simulink subsystem "Out_of_Plane_Model"  (R2025b)
settings: Solver=VariableStepAuto  StartTime=0.0  StopTime=10.0  RelTol=1e-3
undefined symbols (not defined in the file): AeroLiftCff, AeroLongDrgCff, AeroMotoEffctArea, AeroPitchMomentCff, AeroPitchMomentLngth, AeroRltWindAngVect, AeroSideFrcCff, AeroYawMomentCff, aMode, BrkFrntBrkActrBore, BrkFrntBrkActrPrsBpt, BrkFrntBrkPadMeanRadius, BrkFrntBrkTrqTbl, BrkFrntIntrnRadius, BrkFrntKinFricCff, BrkFrntPadNum, BrkFrntShoePinToDrumCntrDst, BrkFrntShoePinToFrcAppDst, BrkFrntShoePinToPadEndAng, BrkFrntShoePinToPadStartAng, BrkFrntStcFricCff, BrkFrntWhlSpdBpt, BrkRearBrkActrBore, BrkRearBrkActrPrsBpt, BrkRearBrkPadMeanRadius, BrkRearBrkTrqTbl, BrkRearIntrnRadius, BrkRearKinFricCff, BrkRearPadNum, BrkRearShoePinToDrumCntrDst, BrkRearShoePinToFrcAppDst, BrkRearShoePinToPadEndAng, BrkRearShoePinToPadStartAng, BrkRearStcFricCff, BrkRearWhlSpdBpt, CpRrVx0, CpRrVy0, CpRrY0, EnvAbsPrs, EnvAirTemp, FrkFrL0, FrmAng0, g, GasCnst, InitFrkLngth, InitMainFrmPitchAng, InitRearArmPitchAng, InitRearCntctPtchLatVel, InitRearCntctPtchLongVel, InitRearCntctPtchZ, InitYawAng, MotoFrmLngth, MotoFrmMass, MotoGrvty, MotoLatOfst, MotoLongOfst, MotoLowrFrntFrkMass, MotoPtchOfst, MotoRearArmLngth, MotoRearArmMass ... (+28)
libraries: sm_lib x309, nesl_utility_internal x158, nesl_utility x7, autolibsharedcoupling x6, vehdynlibtire x6, sharedtransform x4, shared6dof x1, matrix_library x1, vehdynlibeomcommon x1
(part 6 of 10)

== system Out_of_Plane_Model/Chassis, Tires, and Areo/Tire/Front Tire/Linear Front Simscape Tire/Simscape/apply forces and moments ==
  Fx : Inport
  Fy : Inport  Port=2
  Fz : Inport  Port=3
  Mxin : Inport  Port=4
  Mzin : Inport  Port=5
  External Force and Torque : sm_lib/Forces and Torques/External Force and Torque  EnableForceX=on  EnableForceY=on  EnableForceZ=on  EnableForce=off  ForceResolutionFrame=AttachedFrame  EnableTorqueX=on  EnableTorqueY=off  EnableTorqueZ=on  EnableTorque=off  TorqueResolutionFrame=AttachedFrame
  Simulink-PS Converter : nesl_utility_internal/Simulink-PS Converter  PhysicalDomain=network_engine_domain  SubClassName=ps_input  LeftPortType=input  RightPortType=output  PseudoPeriodic=off  Frequencies=[]  NoiseDistribution=none  NoiseParameters=[]  Unit=N  AffineConversion=off  FilteringAndDerivatives=zero  SimscapeFilterOrder=1  InputFilterTimeConstant=0.001  UdotUserProvided=1
  Simulink-PS Converter1 : nesl_utility_internal/Simulink-PS Converter  PhysicalDomain=network_engine_domain  SubClassName=ps_input  LeftPortType=input  RightPortType=output  PseudoPeriodic=off  Frequencies=[]  NoiseDistribution=none  NoiseParameters=[]  Unit=N  AffineConversion=off  FilteringAndDerivatives=zero  SimscapeFilterOrder=1  InputFilterTimeConstant=0.001  UdotUserProvided=1
  Simulink-PS Converter2 : nesl_utility_internal/Simulink-PS Converter  PhysicalDomain=network_engine_domain  SubClassName=ps_input  LeftPortType=input  RightPortType=output  PseudoPeriodic=off  Frequencies=[]  NoiseDistribution=none  NoiseParameters=[]  Unit=N  AffineConversion=off  FilteringAndDerivatives=zero  SimscapeFilterOrder=1  InputFilterTimeConstant=0.001  UdotUserProvided=1
  Simulink-PS Converter3 : nesl_utility_internal/Simulink-PS Converter  PhysicalDomain=network_engine_domain  SubClassName=ps_input  LeftPortType=input  RightPortType=output  PseudoPeriodic=off  Frequencies=[]  NoiseDistribution=none  NoiseParameters=[]  Unit=N*m  AffineConversion=off  FilteringAndDerivatives=zero  SimscapeFilterOrder=1  InputFilterTimeConstant=0.001  UdotUserProvided=1
  Simulink-PS Converter4 : nesl_utility_internal/Simulink-PS Converter  PhysicalDomain=network_engine_domain  SubClassName=ps_input  LeftPortType=input  RightPortType=output  PseudoPeriodic=off  Frequencies=[]  NoiseDistribution=none  NoiseParameters=[]  Unit=N*m  AffineConversion=off  FilteringAndDerivatives=zero  SimscapeFilterOrder=1  InputFilterTimeConstant=0.001  UdotUserProvided=1
  CP : PMIOPort  Side=Right
  wires:
  Fx/1 -> Simulink-PS Converter/1
  Fz/1 -> Simulink-PS Converter2/1
  Fy/1 -> Simulink-PS Converter1/1
  Mxin/1 -> Simulink-PS Converter3/1
  Mzin/1 -> Simulink-PS Converter4/1
  connections:
  External Force and Torque/LConn3 -- Simulink-PS Converter2/RConn1
  External Force and Torque/LConn1 -- Simulink-PS Converter/RConn1
  External Force and Torque/RConn1 -- CP/RConn1
  Simulink-PS Converter1/RConn1 -- External Force and Torque/LConn2
  External Force and Torque/LConn4 -- Simulink-PS Converter3/RConn1
  External Force and Torque/LConn5 -- Simulink-PS Converter4/RConn1

== system Out_of_Plane_Model/Chassis, Tires, and Areo/Tire/Rear Tire/Linear Rear Simscape Tire/Brake model/External ==
  MBrkin : Inport
  MBrk : Outport
  wires:
  MBrkin/1 -> MBrk/1

== system Out_of_Plane_Model/Chassis, Tires, and Areo/Tire/Rear Tire/Linear Rear Simscape Tire/Brake model/MW Brake ==
  BrkPrs : Inport
  Omega : Inport  Port=2
  Brakes : Subsystem  Variant=on  VariantControlMode=label  LabelModeActiveChoice=Disk  mask{aMode=aMode}
  Gain1 : Gain  Gain=4
  Product : Product
  Tanh : Trigonometry  Operator=tanh
  Unary Minus : UnaryMinus
  MBrk : Outport
  wires:
  BrkPrs/1 -> Brakes/1(BrkPrs)
  Unary Minus/1 -> MBrk/1
  Product/1 -> Unary Minus/1
  Omega/1 -> Brakes/2(Omega), Gain1/1
  Tanh/1 -> Product/2
  Brakes/1(MyBrk) -> Product/1
  Gain1/1 -> Tanh/1

== system Out_of_Plane_Model/Chassis, Tires, and Areo/Tire/Rear Tire/Linear Rear Simscape Tire/Contact model/External ==
  Fzin : Inport
  Fz : Outport
  wires:
  Fzin/1 -> Fz/1

== system Out_of_Plane_Model/Chassis, Tires, and Areo/Tire/Rear Tire/Linear Rear Simscape Tire/Contact model/Simple spring and damper ==
  rz : Inport
  pz : Inport  Port=2
  Add4 : Sum
  Gain17 : Gain  Gain=kz
  Gain18 : Gain  Gain=cz
  Unary Minus : UnaryMinus
  contact decision : Subsystem
  Fz : Outport
  wires:
  pz/1 -> Gain17/1, contact decision/1(pos)
  Gain17/1 -> Add4/1
  Add4/1 -> contact decision/2(Fpre)
  contact decision/1(F) -> Unary Minus/1
  Gain18/1 -> Add4/2
  rz/1 -> Gain18/1
  Unary Minus/1 -> Fz/1

== system Out_of_Plane_Model/Chassis, Tires, and Areo/Tire/Rear Tire/Linear Rear Simscape Tire/Friction model/External ==
  rx : Inport
  ry : Inport  Port=2
  rz : Inport  Port=3
  Omega : Inport  Port=4
  Fxin : Inport  Port=5
  Fyin : Inport  Port=6
  Mxin : Inport  Port=7
  Myin : Inport  Port=8
  Mzin : Inport  Port=9
  Calc. part Vertical load & SideSlipAngle : Subsystem
  Mux : Mux  Inputs=3
  SlipRatio : Subsystem
  Fx : Outport
  Fy : Outport  Port=2
  Kappa : Outport  Port=3
  Alpha : Outport  Port=4
  Mx : Outport  Port=5
  My : Outport  Port=6
  Mz : Outport  Port=7
  wires:
  Mzin/1 -> Mz/1
  Mxin/1 -> Mx/1
  Myin/1 -> My/1
  SlipRatio/1(SlipRatio) -> Kappa/1
  Fyin/1 -> Fy/1
  Fxin/1 -> Fx/1
  Mux/1 -> Calc. part Vertical load & SideSlipAngle/1(vel.)
  rx/1 -> Mux/1
  ry/1 -> Mux/2
  rz/1 -> Mux/3
  Calc. part Vertical load & SideSlipAngle/2(SideSlipAngle [rad]) -> Alpha/1
  Calc. part Vertical load & SideSlipAngle/1(Road Vel.) -> SlipRatio/1(RoadVelocity)
  Omega/1 -> SlipRatio/2(Rot.Velocity)

== system Out_of_Plane_Model/Chassis, Tires, and Areo/Tire/Rear Tire/Linear Rear Simscape Tire/Friction model/Linear ==
  rx : Inport
  ry : Inport  Port=2
  rz : Inport  Port=3
  Fz : Inport  Port=4
  Omega : Inport  Port=5
  A,V,P_WhlRoll : Inport  Port=6
  Mxin : Inport  Port=7
  Myin : Inport  Port=8
  Mzin : Inport  Port=9
  Add : Sum  Inputs=--
  Bus Selector : BusSelector  OutputSignals=WhlPRoll
  Camber stiffness : Gain  Gain=kyc
  Cornering stiffness : Gain  Gain=kyl
  Divide1 : Product  Inputs=**
  Divide2 : Product  Inputs=**
  Divide3 : Product  Inputs=**
  Driving/Braking stiffness : Gain  Gain=kx
  Saturation1 : Saturate  UpperLimit=20000  LowerLimit=100  ZeroCross=off
  Slip Angle : vehdynlibtire/Dugoff Wheel 2DOF/Dugoff/Slip Angle  mask{Lrely=.001, ALPMAX=pi, ALPMIN=-pi}
      mask prompts: Lrely "Lateral relaxation length [m]:"; ALPMAX "Max slip angle [rad]:"; ALPMIN "Min slip angle [rad]:"
      settings: LibrarySourceBlock=vehdynlibtire/Fiala Wheel 2DOF/Fiala/Slip Angle
  SlipRatio : Subsystem
  Terminator : Terminator
  Terminator1 : Terminator
  Unary Minus1 : UnaryMinus
  Unary Minus3 : UnaryMinus
  Fx : Outport
  Fy : Outport  Port=2
  Kappa : Outport  Port=3
  Alpha : Outport  Port=4
  Mx : Outport  Port=5
  My : Outport  Port=6
  Mz : Outport  Port=7
  wires:
  Add/1 -> Fy/1  "Fy"
  Slip Angle/1 -> Terminator1/1
  Unary Minus3/1 -> Fx/1  "Fx"
  Divide2/1 -> Add/2  "Fyc"
  Camber stiffness/1 -> Divide2/1
  Bus Selector/1 -> Camber stiffness/1  "<WhlPRoll>"
  A,V,P_WhlRoll/1 -> Bus Selector/1
  Slip Angle/2 -> Cornering stiffness/1, Alpha/1
  Cornering stiffness/1 -> Divide3/1
  rz/1 -> Terminator/1
  Fz/1 -> Unary Minus1/1
  rx/1 -> Slip Angle/1, SlipRatio/1(RoadVelocity)
  Unary Minus1/1 -> Saturation1/1
  SlipRatio/1(SlipRatio) -> Driving/Braking stiffness/1, Kappa/1
  Omega/1 -> SlipRatio/2(Rot.Velocity)
  ry/1 -> Slip Angle/2
  Driving/Braking stiffness/1 -> Divide1/1
  Divide1/1 -> Unary Minus3/1
  Divide3/1 -> Add/1  "Fyl"
  Mxin/1 -> Mx/1
  Myin/1 -> My/1
  Mzin/1 -> Mz/1
  Saturation1/1 -> Divide2/2, Divide1/2, Divide3/2

== system Out_of_Plane_Model/Chassis, Tires, and Areo/Tire/Rear Tire/Linear Rear Simscape Tire/Friction model/LinearOld ==
  rx : Inport
  ry : Inport  Port=2
  rz : Inport  Port=3
  Fz : Inport  Port=4
  Omega : Inport  Port=5
  A,V,P_WhlRoll : Inport  Port=6
  Mxin : Inport  Port=7
  Myin : Inport  Port=8
  Mzin : Inport  Port=9
  Add : Sum
  Bus Selector : BusSelector  OutputSignals=WhlPRoll
  Calc. part Vertical load & SideSlipAngle : Subsystem
  Camber stiffness : Gain  Gain=kyc
  Cornering stiffness : Gain  Gain=kyl
  Divide1 : Product  Inputs=**
  Divide2 : Product  Inputs=**
  Divide3 : Product  Inputs=**
  Driving/Braking stiffness : Gain  Gain=kx
  Mux : Mux  Inputs=3
  SlipRatio : Subsystem
  Unary Minus1 : UnaryMinus
  Unary Minus2 : UnaryMinus
  Unary Minus3 : UnaryMinus
  Fx : Outport
  Fy : Outport  Port=2
  Kappa : Outport  Port=3
  Alpha : Outport  Port=4
  Mx : Outport  Port=5
  My : Outport  Port=6
  Mz : Outport  Port=7
  wires:
  Mzin/1 -> Mz/1
  Myin/1 -> My/1
  Mxin/1 -> Mx/1
  Divide3/1 -> Add/1  "Fyl"
  Divide1/1 -> Unary Minus3/1
  Driving/Braking stiffness/1 -> Divide1/1
  ry/1 -> Mux/2
  Omega/1 -> SlipRatio/3(Rot.Velocity)
  SlipRatio/1(SlipRatio) -> Kappa/1, Driving/Braking stiffness/1
  Unary Minus1/1 -> Divide3/2, Divide1/2, Divide2/2
  rx/1 -> Mux/1
  Fz/1 -> Unary Minus1/1
  rz/1 -> Mux/3
  Cornering stiffness/1 -> Divide3/1
  Calc. part Vertical load & SideSlipAngle/1(Road Vel.) -> SlipRatio/1(RoadVelocity)
  Mux/1 -> Calc. part Vertical load & SideSlipAngle/1(vel.)
  Calc. part Vertical load & SideSlipAngle/2(SideSlipAngle [rad]) -> Cornering stiffness/1, Alpha/1, SlipRatio/2(SlipAngle)
  A,V,P_WhlRoll/1 -> Bus Selector/1
  Bus Selector/1 -> Camber stiffness/1  "<WhlPRoll>"
  Camber stiffness/1 -> Divide2/1
  Divide2/1 -> Unary Minus2/1
  Add/1 -> Fy/1  "Fy"
  Unary Minus2/1 -> Add/2  "Fyc"
  Unary Minus3/1 -> Fx/1  "Fx"

== system Out_of_Plane_Model/Chassis, Tires, and Areo/Tire/Rear Tire/Linear Rear Simscape Tire/Simscape/Reaction Torque ==
  MWh : Inport
  Mbrk : Inport  Port=2
  External Force and Torque1 : sm_lib/Forces and Torques/External Force and Torque  EnableForceX=off  EnableForceY=off  EnableForceZ=off  EnableForce=off  ForceResolutionFrame=World  EnableTorqueX=off  EnableTorqueY=on  EnableTorqueZ=off  EnableTorque=off  TorqueResolutionFrame=AttachedFrame
  Minus1 : Sum  Inputs=--
  Simulink-PS Converter1 : nesl_utility_internal/Simulink-PS Converter  PhysicalDomain=network_engine_domain  SubClassName=ps_input  LeftPortType=input  RightPortType=output  PseudoPeriodic=off  Frequencies=[]  NoiseDistribution=none  NoiseParameters=[]  Unit=1  AffineConversion=off  FilteringAndDerivatives=provide  SimscapeFilterOrder=1  InputFilterTimeConstant=0.001  UdotUserProvided=0
  M : PMIOPort  Side=Right
  wires:
  Minus1/1 -> Simulink-PS Converter1/1
  Mbrk/1 -> Minus1/2
  MWh/1 -> Minus1/1
  connections:
  Simulink-PS Converter1/RConn1 -- External Force and Torque1/LConn1
  External Force and Torque1/RConn1 -- M/RConn1

== system Out_of_Plane_Model/Chassis, Tires, and Areo/Tire/Rear Tire/Linear Rear Simscape Tire/Simscape/Sensor ==
  PS-Simulink Converter{1..2,4..5} (4 alike) : nesl_utility_internal/PS-Simulink Converter  PhysicalDomain=network_engine_domain  SubClassName=ps_output  LeftPortType=input  RightPortType=output  PseudoPeriodic=off  Frequencies=[]  VectorFormat=1-D array  Unit=inherit  AffineConversion=off
  Transform Sensor : sm_lib/Frames and Transforms/Transform Sensor  MeasurementFrame=NonRotatingFollower  RotationSequence=XYX  SenseAngle=off  SenseAxis=off  SenseQ=off  SenseR=off  SenseRotationSequence=off  SenseOmegaX=off  SenseOmegaY=off  SenseOmegaZ=off  SenseOmega=off  SenseQDot=off  SenseRDot=off  SenseRotationSequenceDot=off  SenseAlphaX=off  SenseAlphaY=off  SenseAlphaZ=off  SenseAlpha=off  SenseQDDot=off  SenseRDDot=off  SenseX=off  SenseY=off  SenseZ=on  SenseXYZ=off  SenseRad=off  SenseAzim=off  SenseDist=off  SenseInc=off  SenseXDot=on  SenseYDot=on  SenseZDot=on  SenseXYZDot=off  SenseRadDot=off  SenseAzimDot=off  SenseDistDot=off  SenseIncDot=off  SenseXDDot=off  SenseYDDot=off  SenseZDDot=off  SenseXYZDDot=off  SenseRadDDot=off  SenseAzimDDot=off  SenseDistDDot=off  SenseIncDDot=off
  World Frame : sm_lib/Frames and Transforms/World Frame
  F : PMIOPort  Side=Left
  rx : Outport
  ry : Outport  Port=2
  rz : Outport  Port=3
  pz : Outport  Port=4
  wires:
  PS-Simulink Converter4/1 -> rz/1
  PS-Simulink Converter2/1 -> pz/1
  PS-Simulink Converter5/1 -> rx/1
  PS-Simulink Converter1/1 -> ry/1
  connections:
  Transform Sensor/LConn1 -- World Frame/RConn1
  Transform Sensor/RConn1 -- F/RConn1
  PS-Simulink Converter2/LConn1 -- Transform Sensor/RConn2
  Transform Sensor/RConn3 -- PS-Simulink Converter5/LConn1
  PS-Simulink Converter1/LConn1 -- Transform Sensor/RConn4
  PS-Simulink Converter4/LConn1 -- Transform Sensor/RConn5

== system Out_of_Plane_Model/Chassis, Tires, and Areo/Tire/Rear Tire/Linear Rear Simscape Tire/Simscape/Simscape Multibody Rim&Wheel ==
  MWh : Inport
  Fx : Inport  Port=2
  Mbrk : Inport  Port=3
  Myin : Inport  Port=4
  Mcr : Inport  Port=5
  Add_Torque : Sum  Inputs=+++
  Gain5 : Gain  Gain=RWhl
  Minus2 : Sum  Inputs=+++
  Tire_Rim_wth_transient : Subsystem
  B : PMIOPort  Side=Left
  CP : PMIOPort  Port=2  Side=Right
  omega : Outport
  omegadot : Outport  Port=2
  A,V,P_WhlRoll : Outport  Port=3
  Info_CP : Outport  Port=4
  wires:
  Tire_Rim_wth_transient/4(Info_CP) -> Info_CP/1
  Gain5/1 -> Add_Torque/2
  Tire_Rim_wth_transient/3(A,V,P_WhlRoll) -> A,V,P_WhlRoll/1
  Minus2/1 -> Add_Torque/1
  Mbrk/1 -> Add_Torque/3
  Fx/1 -> Gain5/1
  Mcr/1 -> Minus2/2
  MWh/1 -> Minus2/1
  Add_Torque/1 -> Tire_Rim_wth_transient/1(Ext.F_T)
  Tire_Rim_wth_transient/1(omega) -> omega/1
  Myin/1 -> Minus2/3
  Tire_Rim_wth_transient/2(omegadot) -> omegadot/1
  connections:
  Tire_Rim_wth_transient/LConn1 -- B/RConn1
  CP/RConn1 -- Tire_Rim_wth_transient/LConn2

== system Out_of_Plane_Model/Chassis, Tires, and Areo/Tire/Rear Tire/Linear Rear Simscape Tire/Simscape/apply forces and moments ==
  Fx : Inport
  Fy : Inport  Port=2
  Fz : Inport  Port=3
  Mxin : Inport  Port=4
  Mzin : Inport  Port=5
  External Force and Torque : sm_lib/Forces and Torques/External Force and Torque  EnableForceX=on  EnableForceY=on  EnableForceZ=on  EnableForce=off  ForceResolutionFrame=AttachedFrame  EnableTorqueX=on  EnableTorqueY=off  EnableTorqueZ=on  EnableTorque=off  TorqueResolutionFrame=AttachedFrame
  Simulink-PS Converter : nesl_utility_internal/Simulink-PS Converter  PhysicalDomain=network_engine_domain  SubClassName=ps_input  LeftPortType=input  RightPortType=output  PseudoPeriodic=off  Frequencies=[]  NoiseDistribution=none  NoiseParameters=[]  Unit=N  AffineConversion=off  FilteringAndDerivatives=zero  SimscapeFilterOrder=1  InputFilterTimeConstant=0.001  UdotUserProvided=1
  Simulink-PS Converter1 : nesl_utility_internal/Simulink-PS Converter  PhysicalDomain=network_engine_domain  SubClassName=ps_input  LeftPortType=input  RightPortType=output  PseudoPeriodic=off  Frequencies=[]  NoiseDistribution=none  NoiseParameters=[]  Unit=N  AffineConversion=off  FilteringAndDerivatives=zero  SimscapeFilterOrder=1  InputFilterTimeConstant=0.001  UdotUserProvided=1
  Simulink-PS Converter2 : nesl_utility_internal/Simulink-PS Converter  PhysicalDomain=network_engine_domain  SubClassName=ps_input  LeftPortType=input  RightPortType=output  PseudoPeriodic=off  Frequencies=[]  NoiseDistribution=none  NoiseParameters=[]  Unit=N  AffineConversion=off  FilteringAndDerivatives=zero  SimscapeFilterOrder=1  InputFilterTimeConstant=0.001  UdotUserProvided=1
  Simulink-PS Converter3 : nesl_utility_internal/Simulink-PS Converter  PhysicalDomain=network_engine_domain  SubClassName=ps_input  LeftPortType=input  RightPortType=output  PseudoPeriodic=off  Frequencies=[]  NoiseDistribution=none  NoiseParameters=[]  Unit=N*m  AffineConversion=off  FilteringAndDerivatives=zero  SimscapeFilterOrder=1  InputFilterTimeConstant=0.001  UdotUserProvided=1
  Simulink-PS Converter4 : nesl_utility_internal/Simulink-PS Converter  PhysicalDomain=network_engine_domain  SubClassName=ps_input  LeftPortType=input  RightPortType=output  PseudoPeriodic=off  Frequencies=[]  NoiseDistribution=none  NoiseParameters=[]  Unit=N*m  AffineConversion=off  FilteringAndDerivatives=zero  SimscapeFilterOrder=1  InputFilterTimeConstant=0.001  UdotUserProvided=1
  CP : PMIOPort  Side=Right
  wires:
  Fx/1 -> Simulink-PS Converter/1
  Fz/1 -> Simulink-PS Converter2/1
  Fy/1 -> Simulink-PS Converter1/1
  Mxin/1 -> Simulink-PS Converter3/1
  Mzin/1 -> Simulink-PS Converter4/1
  connections:
  External Force and Torque/LConn3 -- Simulink-PS Converter2/RConn1
  External Force and Torque/LConn1 -- Simulink-PS Converter/RConn1
  External Force and Torque/RConn1 -- CP/RConn1
  Simulink-PS Converter1/RConn1 -- External Force and Torque/LConn2
  External Force and Torque/LConn4 -- Simulink-PS Converter3/RConn1
  External Force and Torque/LConn5 -- Simulink-PS Converter4/RConn1

== system Out_of_Plane_Model/Chassis, Tires, and Areo/Chassis Body, Suspension, and Steering/CHASSIS/Chassis body/CPRr/Camera/Right ==
  base : sm_lib/Body Elements/Graphic  GraphicType=Marker  MarkerShape=Cube  MarkerSize=1  GraphicVisPropType=SimpleVisualProperties  GraphicDiffuseColor=[0.0 0.0 0.0]  GraphicOpacity=1.0  GraphicSpecularColor=[0.5 0.5 0.5 1.0]  GraphicAmbientColor=[0.15 0.15 0.15 1.0]  GraphicEmissiveColor=[0.0 0.0 0.0 1.0]  GraphicShininess=75
  cam : sm_lib/Frames and Transforms/Rigid Transform  RotationMethod=None  FollAlignAxisA=+X  BaseAlignAxisA=+Y  FollAlignAxisB=+Y  BaseAlignAxisB=+Z  RotationStandardAxis=+X  RotationAngle=0  RotationAngleUnits=rad  RotationArbitraryAxis=[0 0 1]  RotationSequenceAxes=FollowerAxes  RotationSequence=XYX  RotationSequenceAngles=[0 0 0]  RotationSequenceAnglesUnits=deg  RotationMatrix=[1 0 0; 0 1 0; 0 0 1]  Quaternion=[1 0 0 0]  TranslationMethod=Cartesian  TranslationCartesianOffset=[1 3 -1]  TranslationCartesianOffsetUnits=m  TranslationStandardAxis=+Z  TranslationStandardOffset=0  TranslationStandardOffsetUnits=m  TranslationROffset=0  TranslationROffsetUnits=m  TranslationThetaOffset=0  TranslationThetaOffsetUnits=deg  TranslationZOffset=0  TranslationZOffsetUnits=m
  cam1 : sm_lib/Frames and Transforms/Rigid Transform  RotationMethod=None  FollAlignAxisA=+X  BaseAlignAxisA=+Y  FollAlignAxisB=+Y  BaseAlignAxisB=+Z  RotationStandardAxis=+X  RotationAngle=0  RotationAngleUnits=rad  RotationArbitraryAxis=[0 0 1]  RotationSequenceAxes=FollowerAxes  RotationSequence=XYX  RotationSequenceAngles=[0 0 0]  RotationSequenceAnglesUnits=deg  RotationMatrix=[1 0 0; 0 1 0; 0 0 1]  Quaternion=[1 0 0 0]  TranslationMethod=Cartesian  TranslationCartesianOffset=[1 0 -1]  TranslationCartesianOffsetUnits=m  TranslationStandardAxis=+Z  TranslationStandardOffset=0  TranslationStandardOffsetUnits=m  TranslationROffset=0  TranslationROffsetUnits=m  TranslationThetaOffset=0  TranslationThetaOffsetUnits=deg  TranslationZOffset=0  TranslationZOffsetUnits=m
  target : sm_lib/Body Elements/Graphic  GraphicType=Marker  MarkerShape=Cube  MarkerSize=1  GraphicVisPropType=SimpleVisualProperties  GraphicDiffuseColor=[0.0 0.0 0.0]  GraphicOpacity=1.0  GraphicSpecularColor=[0.5 0.5 0.5 1.0]  GraphicAmbientColor=[0.15 0.15 0.15 1.0]  GraphicEmissiveColor=[0.0 0.0 0.0 1.0]  GraphicShininess=75
  B : PMIOPort  Side=Left
  connections:
  target/RConn1 -- cam1/RConn1
  B/RConn1 -- cam1/LConn1 -- cam/LConn1
  base/RConn1 -- cam/RConn1

== system Out_of_Plane_Model/Chassis, Tires, and Areo/Chassis Body, Suspension, and Steering/CHASSIS/Chassis body/CPRr/Camera_W/LB ==
  base : sm_lib/Body Elements/Graphic  GraphicType=Marker  MarkerShape=Cube  MarkerSize=1  GraphicVisPropType=SimpleVisualProperties  GraphicDiffuseColor=[0.0 0.0 0.0]  GraphicOpacity=1.0  GraphicSpecularColor=[0.5 0.5 0.5 1.0]  GraphicAmbientColor=[0.15 0.15 0.15 1.0]  GraphicEmissiveColor=[0.0 0.0 0.0 1.0]  GraphicShininess=75
  cam : sm_lib/Frames and Transforms/Rigid Transform  RotationMethod=None  FollAlignAxisA=+X  BaseAlignAxisA=+Y  FollAlignAxisB=+Y  BaseAlignAxisB=+Z  RotationStandardAxis=+X  RotationAngle=0  RotationAngleUnits=rad  RotationArbitraryAxis=[0 0 1]  RotationSequenceAxes=FollowerAxes  RotationSequence=XYX  RotationSequenceAngles=[0 0 0]  RotationSequenceAnglesUnits=deg  RotationMatrix=[1 0 0; 0 1 0; 0 0 1]  Quaternion=[1 0 0 0]  TranslationMethod=Cartesian  TranslationCartesianOffset=[-5 -5 -2]  TranslationCartesianOffsetUnits=m  TranslationStandardAxis=+Z  TranslationStandardOffset=0  TranslationStandardOffsetUnits=m  TranslationROffset=0  TranslationROffsetUnits=m  TranslationThetaOffset=0  TranslationThetaOffsetUnits=deg  TranslationZOffset=0  TranslationZOffsetUnits=m
  cam1 : sm_lib/Frames and Transforms/Rigid Transform  RotationMethod=None  FollAlignAxisA=+X  BaseAlignAxisA=+Y  FollAlignAxisB=+Y  BaseAlignAxisB=+Z  RotationStandardAxis=+X  RotationAngle=0  RotationAngleUnits=rad  RotationArbitraryAxis=[0 0 1]  RotationSequenceAxes=FollowerAxes  RotationSequence=XYX  RotationSequenceAngles=[0 0 0]  RotationSequenceAnglesUnits=deg  RotationMatrix=[1 0 0; 0 1 0; 0 0 1]  Quaternion=[1 0 0 0]  TranslationMethod=Cartesian  TranslationCartesianOffset=[1 0 -0.5]  TranslationCartesianOffsetUnits=m  TranslationStandardAxis=+Z  TranslationStandardOffset=0  TranslationStandardOffsetUnits=m  TranslationROffset=0  TranslationROffsetUnits=m  TranslationThetaOffset=0  TranslationThetaOffsetUnits=deg  TranslationZOffset=0  TranslationZOffsetUnits=m
  target : sm_lib/Body Elements/Graphic  GraphicType=Marker  MarkerShape=Cube  MarkerSize=1  GraphicVisPropType=SimpleVisualProperties  GraphicDiffuseColor=[0.0 0.0 0.0]  GraphicOpacity=1.0  GraphicSpecularColor=[0.5 0.5 0.5 1.0]  GraphicAmbientColor=[0.15 0.15 0.15 1.0]  GraphicEmissiveColor=[0.0 0.0 0.0 1.0]  GraphicShininess=75
  B : PMIOPort  Side=Left
  connections:
  target/RConn1 -- cam1/RConn1
  B/RConn1 -- cam1/LConn1 -- cam/LConn1
  base/RConn1 -- cam/RConn1

== system Out_of_Plane_Model/Chassis, Tires, and Areo/Chassis Body, Suspension, and Steering/CHASSIS/Chassis body/CPRr/Camera_W/Right ==
  base : sm_lib/Body Elements/Graphic  GraphicType=Marker  MarkerShape=Cube  MarkerSize=1  GraphicVisPropType=SimpleVisualProperties  GraphicDiffuseColor=[0.0 0.0 0.0]  GraphicOpacity=1.0  GraphicSpecularColor=[0.5 0.5 0.5 1.0]  GraphicAmbientColor=[0.15 0.15 0.15 1.0]  GraphicEmissiveColor=[0.0 0.0 0.0 1.0]  GraphicShininess=75
  cam : sm_lib/Frames and Transforms/Rigid Transform  RotationMethod=None  FollAlignAxisA=+X  BaseAlignAxisA=+Y  FollAlignAxisB=+Y  BaseAlignAxisB=+Z  RotationStandardAxis=+X  RotationAngle=0  RotationAngleUnits=rad  RotationArbitraryAxis=[0 0 1]  RotationSequenceAxes=FollowerAxes  RotationSequence=XYX  RotationSequenceAngles=[0 0 0]  RotationSequenceAnglesUnits=deg  RotationMatrix=[1 0 0; 0 1 0; 0 0 1]  Quaternion=[1 0 0 0]  TranslationMethod=Cartesian  TranslationCartesianOffset=[1 3 -0.5]  TranslationCartesianOffsetUnits=m  TranslationStandardAxis=+Z  TranslationStandardOffset=0  TranslationStandardOffsetUnits=m  TranslationROffset=0  TranslationROffsetUnits=m  TranslationThetaOffset=0  TranslationThetaOffsetUnits=deg  TranslationZOffset=0  TranslationZOffsetUnits=m
  cam1 : sm_lib/Frames and Transforms/Rigid Transform  RotationMethod=None  FollAlignAxisA=+X  BaseAlignAxisA=+Y  FollAlignAxisB=+Y  BaseAlignAxisB=+Z  RotationStandardAxis=+X  RotationAngle=0  RotationAngleUnits=rad  RotationArbitraryAxis=[0 0 1]  RotationSequenceAxes=FollowerAxes  RotationSequence=XYX  RotationSequenceAngles=[0 0 0]  RotationSequenceAnglesUnits=deg  RotationMatrix=[1 0 0; 0 1 0; 0 0 1]  Quaternion=[1 0 0 0]  TranslationMethod=Cartesian  TranslationCartesianOffset=[1 0 -0.5]  TranslationCartesianOffsetUnits=m  TranslationStandardAxis=+Z  TranslationStandardOffset=0  TranslationStandardOffsetUnits=m  TranslationROffset=0  TranslationROffsetUnits=m  TranslationThetaOffset=0  TranslationThetaOffsetUnits=deg  TranslationZOffset=0  TranslationZOffsetUnits=m
  target : sm_lib/Body Elements/Graphic  GraphicType=Marker  MarkerShape=Cube  MarkerSize=1  GraphicVisPropType=SimpleVisualProperties  GraphicDiffuseColor=[0.0 0.0 0.0]  GraphicOpacity=1.0  GraphicSpecularColor=[0.5 0.5 0.5 1.0]  GraphicAmbientColor=[0.15 0.15 0.15 1.0]  GraphicEmissiveColor=[0.0 0.0 0.0 1.0]  GraphicShininess=75
  B : PMIOPort  Side=Left
  connections:
  base/RConn1 -- cam/RConn1
  cam/LConn1 -- cam1/LConn1 -- B/RConn1
  target/RConn1 -- cam1/RConn1

== system Out_of_Plane_Model/Chassis, Tires, and Areo/Chassis Body, Suspension, and Steering/CHASSIS/Chassis body/CPRr/Roll dof/Roll ==
  PS-Simulink Converter13 : nesl_utility_internal/PS-Simulink Converter  PhysicalDomain=network_engine_domain  SubClassName=ps_output  LeftPortType=input  RightPortType=output  PseudoPeriodic=off  Frequencies=[]  VectorFormat=1-D array  Unit=inherit  AffineConversion=off
  PS-Simulink Converter14 : nesl_utility_internal/PS-Simulink Converter  PhysicalDomain=network_engine_domain  SubClassName=ps_output  LeftPortType=input  RightPortType=output  PseudoPeriodic=off  Frequencies=[]  VectorFormat=1-D array  Unit=inherit  AffineConversion=off
  PS-Simulink Converter15 : nesl_utility_internal/PS-Simulink Converter  PhysicalDomain=network_engine_domain  SubClassName=ps_output  LeftPortType=input  RightPortType=output  PseudoPeriodic=off  Frequencies=[]  VectorFormat=1-D array  Unit=inherit  AffineConversion=off
  Rev : sm_lib/Joints/Revolute Joint  JointMode=Normal  CompositeWrenchDir=FollowerOnBase  CompositeWrenchFrame=BaseFrame  SenseConstraintForce=off  SenseConstraintTorque=off  SenseTotalForce=off  SenseTotalTorque=off  PositionTargetSpecify=on  PositionTargetPriority=High  PositionTargetValue=InitRollAng  PositionTargetValueUnits=rad  VelocityTargetSpecify=on  VelocityTargetPriority=High  VelocityTargetValue=InitRollRate  VelocityTargetValueUnits=rad/s  EquilibriumPosition=0  EquilibriumPositionUnits=rad  SpringStiffness=0  SpringStiffnessUnits=N*m/rad  DampingCoefficient=0  DampingCoefficientUnits=N*m/(rad/s)  LowerLimitSpecify=off  LowerLimitBound=-90  LowerLimitBoundUnits=deg  LowerLimitStiffness=1e4  LowerLimitStiffnessUnits=N*m/deg  LowerLimitDamping=10  LowerLimitDampingUnits=N*m/(deg/s)  LowerLimitTransitionRegionWidth=0.1  LowerLimitTransitionRegionWidthUnits=deg  UpperLimitSpecify=off  UpperLimitBound=90  UpperLimitBoundUnits=deg  UpperLimitStiffness=1e4  UpperLimitStiffnessUnits=N*m/deg  UpperLimitDamping=10  UpperLimitDampingUnits=N*m/(deg/s)  UpperLimitTransitionRegionWidth=0.1  UpperLimitTransitionRegionWidthUnits=deg  TorqueActuationMode=NoTorque  MotionActuationMode=ComputedMotion  SensePosition=on  SenseVelocity=on  SenseAcceleration=on  SenseTorqueForce=off  SenseLowerLimitTorqueForce=off  SenseUpperLimitTorqueForce=off
  Y_-pi/2 : sm_lib/Frames and Transforms/Rigid Transform  RotationMethod=StandardAxis  FollAlignAxisA=+X  BaseAlignAxisA=+Y  FollAlignAxisB=+Y  BaseAlignAxisB=+Z  RotationStandardAxis=+Y  RotationAngle=-pi/2  RotationAngleUnits=rad  RotationArbitraryAxis=[0 0 1]  RotationSequenceAxes=FollowerAxes  RotationSequence=XYX  RotationSequenceAngles=[0 0 0]  RotationSequenceAnglesUnits=deg  RotationMatrix=[1 0 0; 0 1 0; 0 0 1]  Quaternion=[1 0 0 0]  TranslationMethod=None  TranslationCartesianOffset=[0 0 0]  TranslationCartesianOffsetUnits=m  TranslationStandardAxis=+Z  TranslationStandardOffset=0  TranslationStandardOffsetUnits=m  TranslationROffset=0  TranslationROffsetUnits=m  TranslationThetaOffset=0  TranslationThetaOffsetUnits=deg  TranslationZOffset=0  TranslationZOffsetUnits=m
  Y_pi/2 : sm_lib/Frames and Transforms/Rigid Transform  RotationMethod=StandardAxis  FollAlignAxisA=+X  BaseAlignAxisA=+Y  FollAlignAxisB=+Y  BaseAlignAxisB=+Z  RotationStandardAxis=+Y  RotationAngle=pi/2  RotationAngleUnits=rad  RotationArbitraryAxis=[0 0 1]  RotationSequenceAxes=FollowerAxes  RotationSequence=XYX  RotationSequenceAngles=[0 0 0]  RotationSequenceAnglesUnits=deg  RotationMatrix=[1 0 0; 0 1 0; 0 0 1]  Quaternion=[1 0 0 0]  TranslationMethod=None  TranslationCartesianOffset=[0 0 0]  TranslationCartesianOffsetUnits=m  TranslationStandardAxis=+Z  TranslationStandardOffset=0  TranslationStandardOffsetUnits=m  TranslationROffset=0  TranslationROffsetUnits=m  TranslationThetaOffset=0  TranslationThetaOffsetUnits=deg  TranslationZOffset=0  TranslationZOffsetUnits=m
  B : PMIOPort  Side=Left
  F : PMIOPort  Port=2  Side=Right
  q : Outport
  w : Outport  Port=2
  b : Outport  Port=3
  wires:
  PS-Simulink Converter15/1 -> b/1  "RollA"
  PS-Simulink Converter14/1 -> w/1  "RollV"
  PS-Simulink Converter13/1 -> q/1  "RollP"
  connections:
  PS-Simulink Converter15/LConn1 -- Rev/RConn4
  PS-Simulink Converter14/LConn1 -- Rev/RConn3
  Rev/RConn1 -- Y_-pi/2/LConn1
  PS-Simulink Converter13/LConn1 -- Rev/RConn2
  Y_pi/2/LConn1 -- B/RConn1
  Rev/LConn1 -- Y_pi/2/RConn1
  Y_-pi/2/RConn1 -- F/RConn1

== system Out_of_Plane_Model/Chassis, Tires, and Areo/Chassis Body, Suspension, and Steering/CHASSIS/Chassis body/CPRr/Roll dof/Roll locked ==
  Constant : Constant  Value=RollAng0
  Constant1 : Constant  Value=0
  B : PMIOPort  Side=Left
  F : PMIOPort  Port=2  Side=Right
  q : Outport
  w : Outport  Port=2
  b : Outport  Port=3
  wires:
  Constant1/1 -> w/1, b/1
  Constant/1 -> q/1
  connections:
  F/RConn1 -- B/RConn1

== system Out_of_Plane_Model/Chassis, Tires, and Areo/Chassis Body, Suspension, and Steering/CHASSIS/Chassis body/CPRr/XYZ dof/XYZ ==
  Cartesian Joint : sm_lib/Joints/Cartesian Joint  JointMode=Normal  CompositeWrenchDir=FollowerOnBase  CompositeWrenchFrame=BaseFrame  SenseConstraintForce=off  SenseConstraintTorque=off  SenseTotalForce=off  SenseTotalTorque=off  PxPositionTargetSpecify=on  PxPositionTargetPriority=High  PxPositionTargetValue=InitRearCntctPtchX  PxPositionTargetValueUnits=m  PxVelocityTargetSpecify=on  PxVelocityTargetPriority=High  PxVelocityTargetValue=InitRearCntctPtchLongVel*cos(InitYawAng)-InitRearCntctPtchLatVel*sin(InitYawAng)  PxVelocityTargetValueUnits=m/s  PxEquilibriumPosition=0  PxEquilibriumPositionUnits=m  PxSpringStiffness=0  PxSpringStiffnessUnits=N/m  PxDampingCoefficient=0  PxDampingCoefficientUnits=N/(m/s)  PxLowerLimitSpecify=off  PxLowerLimitBound=-1  PxLowerLimitBoundUnits=m  PxLowerLimitStiffness=1e6  PxLowerLimitStiffnessUnits=N/m  PxLowerLimitDamping=1e3  PxLowerLimitDampingUnits=N/(m/s)  PxLowerLimitTransitionRegionWidth=1e-4  PxLowerLimitTransitionRegionWidthUnits=m  PxUpperLimitSpecify=off  PxUpperLimitBound=1  PxUpperLimitBoundUnits=m  PxUpperLimitStiffness=1e6  PxUpperLimitStiffnessUnits=N/m  PxUpperLimitDamping=1e3  PxUpperLimitDampingUnits=N/(m/s)  PxUpperLimitTransitionRegionWidth=1e-4  PxUpperLimitTransitionRegionWidthUnits=m  PxTorqueActuationMode=NoTorque  PxMotionActuationMode=ComputedMotion  PxSensePosition=on  PxSenseVelocity=on  PxSenseAcceleration=on  PxSenseTorqueForce=off  PxSenseLowerLimitTorqueForce=off  PxSenseUpperLimitTorqueForce=off  PyPositionTargetSpecify=on  PyPositionTargetPriority=High  PyPositionTargetValue=InitRearCntctPtchY  PyPositionTargetValueUnits=m  PyVelocityTargetSpecify=on  PyVelocityTargetPriority=High  PyVelocityTargetValue=InitRearCntctPtchLongVel*sin(InitYawAng)+InitRearCntctPtchLatVel*cos(InitYawAng)  PyVelocityTargetValueUnits=m/s  PyEquilibriumPosition=0  PyEquilibriumPositionUnits=m  PySpringStiffness=0  PySpringStiffnessUnits=N/m  PyDampingCoefficient=0  PyDampingCoefficientUnits=N/(m/s)  PyLowerLimitSpecify=off  PyLowerLimitBound=-1  PyLowerLimitBoundUnits=m  PyLowerLimitStiffness=1e6  PyLowerLimitStiffnessUnits=N/m  PyLowerLimitDamping=1e3  PyLowerLimitDampingUnits=N/(m/s)  PyLowerLimitTransitionRegionWidth=1e-4  PyLowerLimitTransitionRegionWidthUnits=m  PyUpperLimitSpecify=off  PyUpperLimitBound=1  PyUpperLimitBoundUnits=m  PyUpperLimitStiffness=1e6  PyUpperLimitStiffnessUnits=N/m  PyUpperLimitDamping=1e3  PyUpperLimitDampingUnits=N/(m/s)  PyUpperLimitTransitionRegionWidth=1e-4  PyUpperLimitTransitionRegionWidthUnits=m  PyTorqueActuationMode=NoTorque  PyMotionActuationMode=ComputedMotion  PySensePosition=on  PySenseVelocity=on  PySenseAcceleration=on  PySenseTorqueForce=off  PySenseLowerLimitTorqueForce=off  PySenseUpperLimitTorqueForce=off  PzPositionTargetSpecify=on  PzPositionTargetPriority=High  PzPositionTargetValue=InitRearCntctPtchZ  PzPositionTargetValueUnits=m  PzVelocityTargetSpecify=on  PzVelocityTargetPriority=High  PzVelocityTargetValue=InitRearCntctPtchVertVel  PzVelocityTargetValueUnits=m/s  PzEquilibriumPosition=0  PzEquilibriumPositionUnits=m  PzSpringStiffness=0  PzSpringStiffnessUnits=N/m  PzDampingCoefficient=0  PzDampingCoefficientUnits=N/(m/s)  PzLowerLimitSpecify=off  PzLowerLimitBound=-1  PzLowerLimitBoundUnits=m  PzLowerLimitStiffness=1e6  PzLowerLimitStiffnessUnits=N/m  PzLowerLimitDamping=1e3  PzLowerLimitDampingUnits=N/(m/s)  PzLowerLimitTransitionRegionWidth=1e-4  PzLowerLimitTransitionRegionWidthUnits=m  PzUpperLimitSpecify=off  PzUpperLimitBound=1  PzUpperLimitBoundUnits=m  PzUpperLimitStiffness=1e6  PzUpperLimitStiffnessUnits=N/m  PzUpperLimitDamping=1e3  PzUpperLimitDampingUnits=N/(m/s)  PzUpperLimitTransitionRegionWidth=1e-4  PzUpperLimitTransitionRegionWidthUnits=m  PzTorqueActuationMode=NoTorque  PzMotionActuationMode=ComputedMotion  PzSensePosition=on  PzSenseVelocity=on  PzSenseAcceleration=on  PzSenseTorqueForce=off  PzSenseLowerLimitTorqueForce=off  PzSenseUpperLimitTorqueForce=off
  PS-Simulink Converter{,1..8} (9 alike) : nesl_utility_internal/PS-Simulink Converter  PhysicalDomain=network_engine_domain  SubClassName=ps_output  LeftPortType=input  RightPortType=output  PseudoPeriodic=off  Frequencies=[]  VectorFormat=1-D array  Unit=inherit  AffineConversion=off
  B : PMIOPort  Side=Left
  F : PMIOPort  Port=2  Side=Right
  px : Outport
  vx : Outport  Port=2
  ax : Outport  Port=3
  pz : Outport  Port=4
  vz : Outport  Port=5
  az : Outport  Port=6
  py : Outport  Port=7
  vy : Outport  Port=8
  ay : Outport  Port=9
  wires:
  PS-Simulink Converter8/1 -> az/1
  PS-Simulink Converter7/1 -> vz/1
  PS-Simulink Converter6/1 -> pz/1
  PS-Simulink Converter5/1 -> ay/1
  PS-Simulink Converter4/1 -> vy/1
  PS-Simulink Converter3/1 -> py/1
  PS-Simulink Converter2/1 -> ax/1
  PS-Simulink Converter1/1 -> vx/1
  PS-Simulink Converter/1 -> px/1
  connections:
  Cartesian Joint/RConn10 -- PS-Simulink Converter8/LConn1
  Cartesian Joint/RConn9 -- PS-Simulink Converter7/LConn1
  Cartesian Joint/RConn8 -- PS-Simulink Converter6/LConn1
  Cartesian Joint/RConn7 -- PS-Simulink Converter5/LConn1
  Cartesian Joint/RConn6 -- PS-Simulink Converter4/LConn1
  Cartesian Joint/RConn5 -- PS-Simulink Converter3/LConn1
  Cartesian Joint/RConn4 -- PS-Simulink Converter2/LConn1
  PS-Simulink Converter1/LConn1 -- Cartesian Joint/RConn3
  Cartesian Joint/RConn2 -- PS-Simulink Converter/LConn1
  Cartesian Joint/LConn1 -- B/RConn1
  Cartesian Joint/RConn1 -- F/RConn1

== system Out_of_Plane_Model/Chassis, Tires, and Areo/Chassis Body, Suspension, and Steering/CHASSIS/Chassis body/CPRr/XYZ dof/Y locked ==
  Constant : Constant  Value=CpRrY0
  Constant1 : Constant  Value=0
  PS-Simulink Converter{,1..5} (6 alike) : nesl_utility_internal/PS-Simulink Converter  PhysicalDomain=network_engine_domain  SubClassName=ps_output  LeftPortType=input  RightPortType=output  PseudoPeriodic=off  Frequencies=[]  VectorFormat=1-D array  Unit=inherit  AffineConversion=off
  Rectangular Joint : sm_lib/Joints/Rectangular Joint  JointMode=Normal  CompositeWrenchDir=FollowerOnBase  CompositeWrenchFrame=BaseFrame  SenseConstraintForce=off  SenseConstraintTorque=off  SenseTotalForce=off  SenseTotalTorque=off  PxPositionTargetSpecify=on  PxPositionTargetPriority=High  PxPositionTargetValue=CpRrX0  PxPositionTargetValueUnits=m  PxVelocityTargetSpecify=on  PxVelocityTargetPriority=High  PxVelocityTargetValue=CpRrVx0*cos(YawAng0)-CpRrVy0*sin(YawAng0)  PxVelocityTargetValueUnits=m/s  PxEquilibriumPosition=0  PxEquilibriumPositionUnits=m  PxSpringStiffness=0  PxSpringStiffnessUnits=N/m  PxDampingCoefficient=0  PxDampingCoefficientUnits=N/(m/s)  PxLowerLimitSpecify=off  PxLowerLimitBound=-1  PxLowerLimitBoundUnits=m  PxLowerLimitStiffness=1e6  PxLowerLimitStiffnessUnits=N/m  PxLowerLimitDamping=1e3  PxLowerLimitDampingUnits=N/(m/s)  PxLowerLimitTransitionRegionWidth=1e-4  PxLowerLimitTransitionRegionWidthUnits=m  PxUpperLimitSpecify=off  PxUpperLimitBound=1  PxUpperLimitBoundUnits=m  PxUpperLimitStiffness=1e6  PxUpperLimitStiffnessUnits=N/m  PxUpperLimitDamping=1e3  PxUpperLimitDampingUnits=N/(m/s)  PxUpperLimitTransitionRegionWidth=1e-4  PxUpperLimitTransitionRegionWidthUnits=m  PxTorqueActuationMode=NoTorque  PxMotionActuationMode=ComputedMotion  PxSensePosition=on  PxSenseVelocity=on  PxSenseAcceleration=on  PxSenseTorqueForce=off  PxSenseLowerLimitTorqueForce=off  PxSenseUpperLimitTorqueForce=off  PyPositionTargetSpecify=on  PyPositionTargetPriority=High  PyPositionTargetValue=CpRrZ0  PyPositionTargetValueUnits=m  PyVelocityTargetSpecify=on  PyVelocityTargetPriority=High  PyVelocityTargetValue=CpRrVz0  PyVelocityTargetValueUnits=m/s  PyEquilibriumPosition=0  PyEquilibriumPositionUnits=m  PySpringStiffness=0  PySpringStiffnessUnits=N/m  PyDampingCoefficient=0  PyDampingCoefficientUnits=N/(m/s)  PyLowerLimitSpecify=off  PyLowerLimitBound=-1  PyLowerLimitBoundUnits=m  PyLowerLimitStiffness=1e6  PyLowerLimitStiffnessUnits=N/m  PyLowerLimitDamping=1e3  PyLowerLimitDampingUnits=N/(m/s)  PyLowerLimitTransitionRegionWidth=1e-4  PyLowerLimitTransitionRegionWidthUnits=m  PyUpperLimitSpecify=off  PyUpperLimitBound=1  PyUpperLimitBoundUnits=m  PyUpperLimitStiffness=1e6  PyUpperLimitStiffnessUnits=N/m  PyUpperLimitDamping=1e3  PyUpperLimitDampingUnits=N/(m/s)  PyUpperLimitTransitionRegionWidth=1e-4  PyUpperLimitTransitionRegionWidthUnits=m  PyTorqueActuationMode=NoTorque  PyMotionActuationMode=ComputedMotion  PySensePosition=on  PySenseVelocity=on  PySenseAcceleration=on  PySenseTorqueForce=off  PySenseLowerLimitTorqueForce=off  PySenseUpperLimitTorqueForce=off
  x_-pi/2 : sm_lib/Frames and Transforms/Rigid Transform  RotationMethod=StandardAxis  FollAlignAxisA=+X  BaseAlignAxisA=+Y  FollAlignAxisB=+Y  BaseAlignAxisB=+Z  RotationStandardAxis=+X  RotationAngle=-pi/2  RotationAngleUnits=rad  RotationArbitraryAxis=[0 0 1]  RotationSequenceAxes=FollowerAxes  RotationSequence=XYX  RotationSequenceAngles=[0 0 0]  RotationSequenceAnglesUnits=deg  RotationMatrix=[1 0 0; 0 1 0; 0 0 1]  Quaternion=[1 0 0 0]  TranslationMethod=None  TranslationCartesianOffset=[0 0 0]  TranslationCartesianOffsetUnits=m  TranslationStandardAxis=+Z  TranslationStandardOffset=0  TranslationStandardOffsetUnits=m  TranslationROffset=0  TranslationROffsetUnits=m  TranslationThetaOffset=0  TranslationThetaOffsetUnits=deg  TranslationZOffset=0  TranslationZOffsetUnits=m
  x_pi/2 : sm_lib/Frames and Transforms/Rigid Transform  RotationMethod=StandardAxis  FollAlignAxisA=+X  BaseAlignAxisA=+Y  FollAlignAxisB=+Y  BaseAlignAxisB=+Z  RotationStandardAxis=+X  RotationAngle=pi/2  RotationAngleUnits=rad  RotationArbitraryAxis=[0 0 1]  RotationSequenceAxes=FollowerAxes  RotationSequence=XYX  RotationSequenceAngles=[0 0 0]  RotationSequenceAnglesUnits=deg  RotationMatrix=[1 0 0; 0 1 0; 0 0 1]  Quaternion=[1 0 0 0]  TranslationMethod=None  TranslationCartesianOffset=[0 0 0]  TranslationCartesianOffsetUnits=m  TranslationStandardAxis=+Z  TranslationStandardOffset=0  TranslationStandardOffsetUnits=m  TranslationROffset=0  TranslationROffsetUnits=m  TranslationThetaOffset=0  TranslationThetaOffsetUnits=deg  TranslationZOffset=0  TranslationZOffsetUnits=m
  B : PMIOPort  Side=Left
  F : PMIOPort  Port=2  Side=Right
  px : Outport
  vx : Outport  Port=2
  ax : Outport  Port=3
  pz : Outport  Port=4
  vz : Outport  Port=5
  az : Outport  Port=6
  py : Outport  Port=7
  vy : Outport  Port=8
  ay : Outport  Port=9
  wires:
  Constant1/1 -> vy/1, ay/1
  Constant/1 -> py/1
  PS-Simulink Converter5/1 -> az/1
  PS-Simulink Converter4/1 -> vz/1
  PS-Simulink Converter3/1 -> pz/1
  PS-Simulink Converter2/1 -> ax/1
  PS-Simulink Converter1/1 -> vx/1
  PS-Simulink Converter/1 -> px/1
  connections:
  PS-Simulink Converter5/LConn1 -- Rectangular Joint/RConn7
  PS-Simulink Converter4/LConn1 -- Rectangular Joint/RConn6
  PS-Simulink Converter3/LConn1 -- Rectangular Joint/RConn5
  PS-Simulink Converter2/LConn1 -- Rectangular Joint/RConn4
  Rectangular Joint/RConn3 -- PS-Simulink Converter1/LConn1
  PS-Simulink Converter/LConn1 -- Rectangular Joint/RConn2
  F/RConn1 -- x_-pi/2/RConn1
  B/RConn1 -- x_pi/2/LConn1
  x_-pi/2/LConn1 -- Rectangular Joint/RConn1
  x_pi/2/RConn1 -- Rectangular Joint/LConn1

== system Out_of_Plane_Model/Chassis, Tires, and Areo/Chassis Body, Suspension, and Steering/CHASSIS/Chassis body/CPRr/Yaw dof/Yaw ==
  PS-Simulink Converter13 : nesl_utility_internal/PS-Simulink Converter  PhysicalDomain=network_engine_domain  SubClassName=ps_output  LeftPortType=input  RightPortType=output  PseudoPeriodic=off  Frequencies=[]  VectorFormat=1-D array  Unit=inherit  AffineConversion=off
  PS-Simulink Converter14 : nesl_utility_internal/PS-Simulink Converter  PhysicalDomain=network_engine_domain  SubClassName=ps_output  LeftPortType=input  RightPortType=output  PseudoPeriodic=off  Frequencies=[]  VectorFormat=1-D array  Unit=inherit  AffineConversion=off
  PS-Simulink Converter15 : nesl_utility_internal/PS-Simulink Converter  PhysicalDomain=network_engine_domain  SubClassName=ps_output  LeftPortType=input  RightPortType=output  PseudoPeriodic=off  Frequencies=[]  VectorFormat=1-D array  Unit=inherit  AffineConversion=off
  Yaw dof : sm_lib/Joints/Revolute Joint  JointMode=Normal  CompositeWrenchDir=FollowerOnBase  CompositeWrenchFrame=BaseFrame  SenseConstraintForce=off  SenseConstraintTorque=off  SenseTotalForce=off  SenseTotalTorque=off  PositionTargetSpecify=on  PositionTargetPriority=High  PositionTargetValue=InitYawAng  PositionTargetValueUnits=rad  VelocityTargetSpecify=on  VelocityTargetPriority=High  VelocityTargetValue=InitYawRate  VelocityTargetValueUnits=rad/s  EquilibriumPosition=0  EquilibriumPositionUnits=rad  SpringStiffness=0  SpringStiffnessUnits=N*m/rad  DampingCoefficient=0  DampingCoefficientUnits=N*m/(rad/s)  LowerLimitSpecify=off  LowerLimitBound=-90  LowerLimitBoundUnits=deg  LowerLimitStiffness=1e4  LowerLimitStiffnessUnits=N*m/deg  LowerLimitDamping=10  LowerLimitDampingUnits=N*m/(deg/s)  LowerLimitTransitionRegionWidth=0.1  LowerLimitTransitionRegionWidthUnits=deg  UpperLimitSpecify=off  UpperLimitBound=90  UpperLimitBoundUnits=deg  UpperLimitStiffness=1e4  UpperLimitStiffnessUnits=N*m/deg  UpperLimitDamping=10  UpperLimitDampingUnits=N*m/(deg/s)  UpperLimitTransitionRegionWidth=0.1  UpperLimitTransitionRegionWidthUnits=deg  TorqueActuationMode=NoTorque  MotionActuationMode=ComputedMotion  SensePosition=on  SenseVelocity=on  SenseAcceleration=on  SenseTorqueForce=off  SenseLowerLimitTorqueForce=off  SenseUpperLimitTorqueForce=off
  B : PMIOPort  Side=Left
  F : PMIOPort  Port=2  Side=Right
  q : Outport
  w : Outport  Port=2
  b : Outport  Port=3
  wires:
  PS-Simulink Converter13/1 -> q/1  "RollP"
  PS-Simulink Converter14/1 -> w/1  "RollV"
  PS-Simulink Converter15/1 -> b/1  "RollA"
  connections:
  Yaw dof/RConn1 -- F/RConn1
  B/RConn1 -- Yaw dof/LConn1
  Yaw dof/RConn2 -- PS-Simulink Converter13/LConn1
  Yaw dof/RConn3 -- PS-Simulink Converter14/LConn1
  Yaw dof/RConn4 -- PS-Simulink Converter15/LConn1

== system Out_of_Plane_Model/Chassis, Tires, and Areo/Chassis Body, Suspension, and Steering/CHASSIS/Chassis body/CPRr/Yaw dof/Yaw locked ==
  Constant : Constant  Value=YawAng0
  Constant1 : Constant  Value=0
  B : PMIOPort  Side=Left
  F : PMIOPort  Port=2  Side=Right
  q : Outport
  w : Outport  Port=2
  b : Outport  Port=3
  wires:
  Constant/1 -> q/1
  Constant1/1 -> b/1, w/1
  connections:
  F/RConn1 -- B/RConn1

== system Out_of_Plane_Model/Chassis, Tires, and Areo/Chassis Body, Suspension, and Steering/CHASSIS/Chassis body/Origin&Env/Course shape/none ==

== system Out_of_Plane_Model/Chassis, Tires, and Areo/Chassis Body, Suspension, and Steering/CHASSIS/Chassis body/Origin&Env/Course shape/spline ==
  Spline1 : sm_lib/Curves and Surfaces/Spline  DataPoints=trackData'  DataPointsUnits=m  EndConditionType=Natural  GraphicType=FromGeometry  MarkerShape=Sphere  MarkerSize=10  GraphicVisPropType=SimpleVisualProperties  GraphicDiffuseColor=[0 1 0]  GraphicOpacity=1.0  GraphicSpecularColor=[0.5 0.5 0.5 1.0]  GraphicAmbientColor=[0.15 0.15 0.15 1.0]  GraphicEmissiveColor=[0.0 0.0 0.0 1.0]  GraphicShininess=75
  Spline2 : sm_lib/Curves and Surfaces/Spline  Commented=on  DataPoints=trackData'  DataPointsUnits=m  EndConditionType=Closed  GraphicType=FromGeometry  MarkerShape=Sphere  MarkerSize=10  GraphicVisPropType=SimpleVisualProperties  GraphicDiffuseColor=[0 1 0]  GraphicOpacity=1.0  GraphicSpecularColor=[0.5 0.5 0.5 1.0]  GraphicAmbientColor=[0.15 0.15 0.15 1.0]  GraphicEmissiveColor=[0.0 0.0 0.0 1.0]  GraphicShininess=75
  B : PMIOPort  Side=Left
  connections:
  Spline1/LConn1 -- B/RConn1
